simulink model "Pitch_Attitude_Hold"  (R2024b)
settings: Solver=VariableStepAuto  StartTime=0.0  StopTime=35  RelTol=1e-3
undefined symbols (not defined in the file or in its folder): Ki_2, Kp_1, Kp_2
libraries: slpidlib x2
settings Model: Creator=GH-X-ST  LastModifiedBy=GH-X-ST

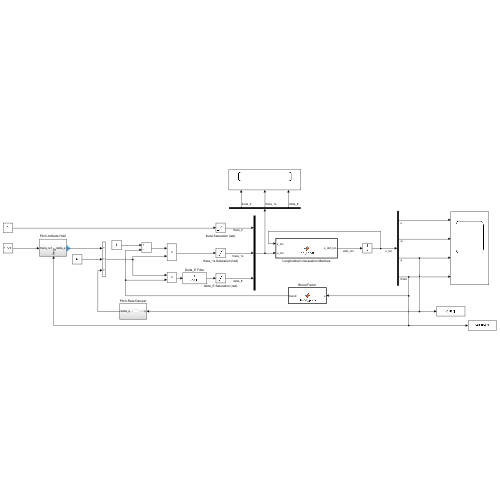
[thumbnail: Simulink's stored preview of the top-level diagram]
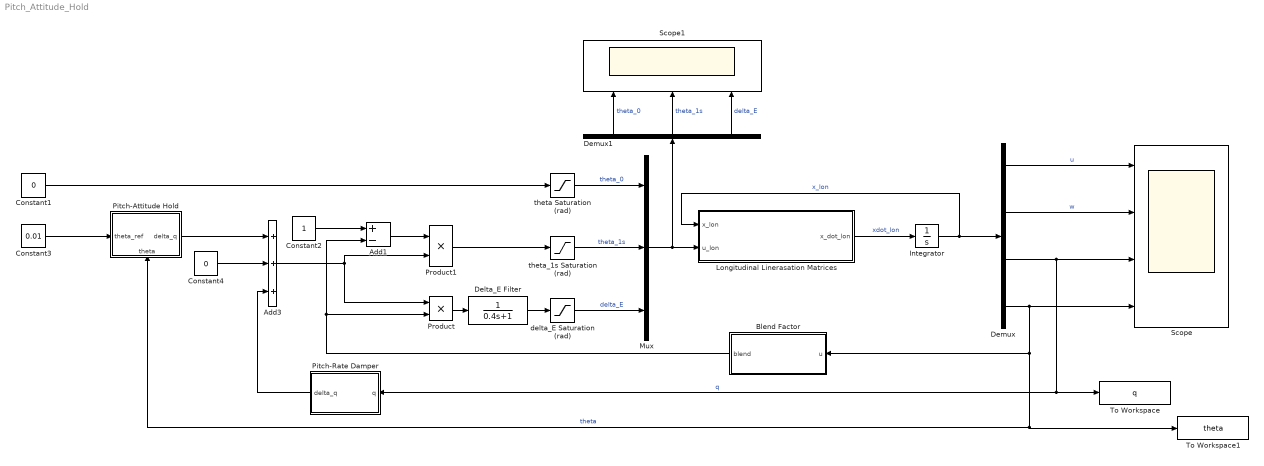
== system Pitch_Attitude_Hold ==
  Add1 : Sum  Inputs=+-
  Add3 : Sum  Inputs=+++
  Blend Factor : MATLAB Function  TreatAsAtomicUnit=on
  Constant1 : Constant  Value=0
  Constant2 : Constant
  Constant3 : Constant  Value=0.01
  Constant4 : Constant  Value=0
  Delta_E Filter : TransferFcn  Denominator=[0.4 1]
  Demux : Demux
  Demux1 : Demux  Outputs=3
  Integrator : Integrator  InitialCondition=[0; 0; 0; 0]
  Longitudinal Linerasation Matrices : MATLAB Function  TreatAsAtomicUnit=on
  Mux : Mux  Inputs=3
  Pitch-Attitude Hold : Subsystem
      settings: PortSchema="{\"entries\":[{\"content\":{\"sides\":[{\"content\":{\"connectorIds\":[\"In1\"]},\"type\":\"ConnectorPlacement.EquallySpacedRectSide\",\"uuid\":\"6ee333b9-9b69-42fd-975a-4580f9624540\"},{\"content\":{\"connectorIds\":[\"Out1\"],\"side\":\"RIGHT\"},\"type\":\"ConnectorPlacement.EquallySpacedRectSide\",\"uuid\":\"6a43d978-a0a5-4636-bfdb-b097e996a039\"},{\"content\":{\"side\":\"TOP\"},\"type\":\"ConnectorPlacement.EquallySpacedRectSide\",\"uuid\":\"00f937d1-ecc9-42d4-adf8-d8f1b79c75a6\"},{\"content\":{\"connectorIds\":[\"In2\"],\"side\":\"BOTTOM\"},\"type\":\"ConnectorPlacement.EquallySpacedRectSide\",\"uuid\":\"809403f9-594f-4491-8a7d-ee0f8643f57e\"}]},\"type\":\"ConnectorPlacement.EquallySpacedConnector\",\"uuid\":\"362aafbc-ebc0-4bb3-8c4e-be284a8bc83f\"}],\"packageUris\":[\"http://schema.mathworks.com/mf0/Connector/R2020b\"],\"version\":\"1.0\"}"
  Pitch-Rate Damper : Subsystem
  Product : Product
  Product1 : Product
  Scope : Scope  NumInputPorts=4
  Scope1 : Scope  NumInputPorts=3
  To Workspace : ToWorkspace  VariableName=q  SaveFormat=Timeseries  SampleTime=-1
  To Workspace1 : ToWorkspace  VariableName=theta  SaveFormat=Timeseries  SampleTime=-1
  delta_E Saturation (rad) : Saturate  UpperLimit=deg2rad(11)  LowerLimit=deg2rad(-11)
  theta Saturation (rad) : Saturate  UpperLimit=deg2rad(20)  LowerLimit=0
  theta_1s Saturation (rad) : Saturate  UpperLimit=deg2rad(6)  LowerLimit=deg2rad(-6)
  wires:
  Longitudinal Linerasation Matrices/1(x_dot_lon) -> Integrator/1  "xdot_lon"
  Integrator/1 -> Longitudinal Linerasation Matrices/1(x_lon), Demux/1  "x_lon"
  Demux/1 -> Scope/1  "u"
  Demux/2 -> Scope/2  "w"
  Demux/3 -> Scope/3, To Workspace/1, Pitch-Rate Damper/1(q)  "q"
  Demux/4 -> To Workspace1/1, Pitch-Attitude Hold/2(theta), Blend Factor/1(u), Scope/4  "theta"
  theta Saturation (rad)/1 -> Mux/1  "theta_0"
  theta_1s Saturation (rad)/1 -> Mux/2  "theta_1s"
  delta_E Saturation (rad)/1 -> Mux/3  "delta_E"
  Blend Factor/1(blend) -> Add1/2, Product/2
  Constant4/1 -> Add3/2
  Pitch-Attitude Hold/1(delta_q) -> Add3/1
  Pitch-Rate Damper/1(delta_q) -> Add3/3
  Add3/1 -> Product/1, Product1/2
  Constant2/1 -> Add1/1
  Add1/1 -> Product1/1
  Mux/1 -> Demux1/1, Longitudinal Linerasation Matrices/2(u_lon)
  Demux1/3 -> Scope1/3  "delta_E"
  Demux1/2 -> Scope1/2  "theta_1s"
  Demux1/1 -> Scope1/1  "theta_0"
  Product/1 -> Delta_E Filter/1
  Product1/1 -> theta_1s Saturation (rad)/1
  Constant1/1 -> theta Saturation (rad)/1
  Constant3/1 -> Pitch-Attitude Hold/1(theta_ref)
  Delta_E Filter/1 -> delta_E Saturation (rad)/1

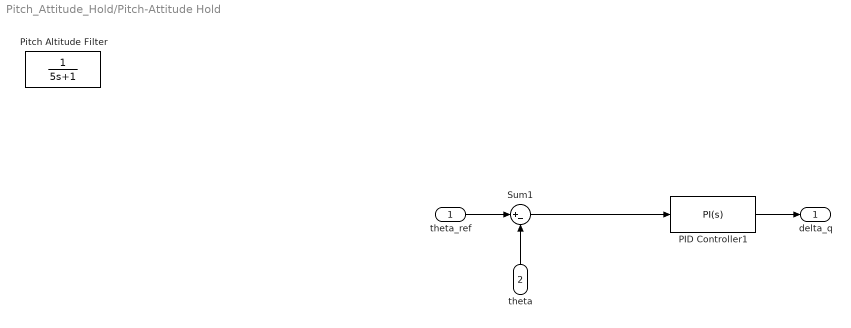
== system Pitch_Attitude_Hold/Pitch-Attitude Hold ==
  theta_ref : Inport
  theta : Inport  Port=2
  PID Controller1 : slpidlib/PID Controller  Controller=PI  Form=Parallel  TimeDomain=Continuous-time  UseExternalTs=off  SampleTime=-1  IntegratorMethod=Forward Euler  FilterMethod=Forward Euler  ControllerParametersSource=internal  P=Kp_2  I=Ki_2  UseKiTs=off  D=0.005  UseExternalDerivativeSource=on  N=100  UseFilter=on  TunerSelectOption=Transfer Function Based (PID Tuner App)  InitialConditionSource=internal  InitialConditionForIntegrator=0  InitialConditionForFilter=0  DifferentiatorICPrevScaledInput=0  ExternalReset=none  TrackingMode=off  Kt=1  LimitOutput=on  SatLimitsSource=internal  UpperSaturationLimit=1  LowerSaturationLimit=-1  LinearizeAsGain=on  AntiWindupMode=none  Kb=1  LimitIntegrator=off  UpperIntegratorSaturationLimit=inf  LowerIntegratorSaturationLimit=-inf  POutMin=[]  POutMax=[]  IOutMin=[]  IOutMax=[]  DOutMin=[]  DOutMax=[]  NOutMin=[]  NOutMax=[]  SumOutMin=[]  SumOutMax=[]  SaturationOutMin=[]  SaturationOutMax=[]  PParamMin=[]  PParamMax=[]  IParamMin=[]  IParamMax=[]  DParamMin=[]  DParamMax=[]  NParamMin=[]  NParamMax=[]  KbParamMin=[]  KbParamMax=[]  KtParamMin=[]  KtParamMax=[]  KbOutMin=[]  KbOutMax=[]  KtOutMin=[]  KtOutMax=[]  IntegratorOutMin=[]  IntegratorOutMax=[]  FilterOutMin=[]  FilterOutMax=[]  SumI1OutMin=[]  SumI1OutMax=[]  SumI2OutMin=[]  SumI2OutMax=[]  SumI3OutMin=[]  SumI3OutMax=[]  SumI4OutMin=[]  SumI4OutMax=[]  SumDOutMin=[]  SumDOutMax=[]  DifferentiatorOutMin=[]  DifferentiatorOutMax=[]  FilterDiffOutCoefMin=[]  FilterDiffOutCoefMax=[]  ReciprocalOutMin=[]  ReciprocalOutMax=[]  SumDenOutMin=[]  SumDenOutMax=[]  SumNumOutMin=[]  SumNumOutMax=[]  DivideOutMin=[]  DivideOutMax=[]  UdiffTsProdOutMin=[]  UdiffTsProdOutMax=[]  NTsProdOutMin=[]  NTsProdOutMax=[]  UintegralTsProdOutMin=[]  UintegralTsProdOutMax=[]  UngainTsProdOutMin=[]  UngainTsProdOutMax=[]  ClampingZeroOutDataTypeStr=Inherit: Inherit via back propagation  ClampingZeroOutMin=[]  ClampingZeroOutMax=[]  FilterDenConstantOutDataTypeStr=Inherit: Inherit via back propagation  FilterDenConstantOutMin=[]  FilterDenConstantOutMax=[]  PCopyOutDataTypeStr=Inherit: Inherit via back propagation  PCopyOutMin=[]  PCopyOutMax=[]  NCopyOutDataTypeStr=Inherit: Inherit via back propagation  NCopyOutMin=[]  NCopyOutMax=[]  IntegratorContinuousStateAttributes=''  IntegratorStateMustResolveToSignalObject=off  IntegratorRTWStateStorageClass=Auto  FilterContinuousStateAttributes=''  FilterStateMustResolveToSignalObject=off  FilterRTWStateStorageClass=Auto  ParallelPVariant=InternalParameters  IdealPVariant=Disabled  IVariant=InternalParameters  DVariant=Disabled  IntegratorVariant=Continuous  SatVariant=Enabled  AWVariant=Passthrough  PCopyVariant=Disabled  TRVariant=Disabled  FdbkBlocksVariant=Forward  IdealPFdbkVariant=Disabled  SatFdbkVariant=Disabled  DerivativeFilterVariant=Disabled  NVariant=Passthrough  NCopyVariant=Disabled_SignalSpec  FilterICVariant=Disabled  IntegratorICVariant=InternalICs  ExternalResetVariant=Disabled  TRSumVariant=Passthrough  SumFdbkVariant=Disabled  SumVariant=Sum_PI  TsampFilterVariant=InternalTs  TsampNgainVariant=Passthrough  TsampIntegralVariant=Disabled_SignalSpec  ExternalSaturationOutDataTypeStr=Inherit: Same as second input  DerivativeSourceVariant=Disabled  PreIntVariant=InternalPreInt
  Pitch Altitude Filter : TransferFcn  Denominator=[5 1]
  Sum1 : Sum  Inputs=|+-
  delta_q : Outport
  wires:
  PID Controller1/1 -> delta_q/1
  theta_ref/1 -> Sum1/1
  theta/1 -> Sum1/2
  Sum1/1 -> PID Controller1/1

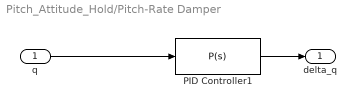
== system Pitch_Attitude_Hold/Pitch-Rate Damper ==
  q : Inport
  PID Controller1 : slpidlib/PID Controller  Controller=P  Form=Parallel  TimeDomain=Continuous-time  UseExternalTs=off  SampleTime=-1  IntegratorMethod=Forward Euler  FilterMethod=Forward Euler  ControllerParametersSource=internal  P=Kp_1  I=0.005  UseKiTs=off  D=0.005  UseExternalDerivativeSource=on  N=100  UseFilter=on  TunerSelectOption=Transfer Function Based (PID Tuner App)  InitialConditionSource=internal  InitialConditionForIntegrator=0  InitialConditionForFilter=0  DifferentiatorICPrevScaledInput=0  ExternalReset=none  TrackingMode=off  Kt=1  LimitOutput=on  SatLimitsSource=internal  UpperSaturationLimit=1  LowerSaturationLimit=-1  LinearizeAsGain=on  AntiWindupMode=none  Kb=1  LimitIntegrator=off  UpperIntegratorSaturationLimit=inf  LowerIntegratorSaturationLimit=-inf  POutMin=[]  POutMax=[]  IOutMin=[]  IOutMax=[]  DOutMin=[]  DOutMax=[]  NOutMin=[]  NOutMax=[]  SumOutMin=[]  SumOutMax=[]  SaturationOutMin=[]  SaturationOutMax=[]  PParamMin=[]  PParamMax=[]  IParamMin=[]  IParamMax=[]  DParamMin=[]  DParamMax=[]  NParamMin=[]  NParamMax=[]  KbParamMin=[]  KbParamMax=[]  KtParamMin=[]  KtParamMax=[]  KbOutMin=[]  KbOutMax=[]  KtOutMin=[]  KtOutMax=[]  IntegratorOutMin=[]  IntegratorOutMax=[]  FilterOutMin=[]  FilterOutMax=[]  SumI1OutMin=[]  SumI1OutMax=[]  SumI2OutMin=[]  SumI2OutMax=[]  SumI3OutMin=[]  SumI3OutMax=[]  SumI4OutMin=[]  SumI4OutMax=[]  SumDOutMin=[]  SumDOutMax=[]  DifferentiatorOutMin=[]  DifferentiatorOutMax=[]  FilterDiffOutCoefMin=[]  FilterDiffOutCoefMax=[]  ReciprocalOutMin=[]  ReciprocalOutMax=[]  SumDenOutMin=[]  SumDenOutMax=[]  SumNumOutMin=[]  SumNumOutMax=[]  DivideOutMin=[]  DivideOutMax=[]  UdiffTsProdOutMin=[]  UdiffTsProdOutMax=[]  NTsProdOutMin=[]  NTsProdOutMax=[]  UintegralTsProdOutMin=[]  UintegralTsProdOutMax=[]  UngainTsProdOutMin=[]  UngainTsProdOutMax=[]  ClampingZeroOutDataTypeStr=Inherit: Inherit via back propagation  ClampingZeroOutMin=[]  ClampingZeroOutMax=[]  FilterDenConstantOutDataTypeStr=Inherit: Inherit via back propagation  FilterDenConstantOutMin=[]  FilterDenConstantOutMax=[]  PCopyOutDataTypeStr=Inherit: Inherit via back propagation  PCopyOutMin=[]  PCopyOutMax=[]  NCopyOutDataTypeStr=Inherit: Inherit via back propagation  NCopyOutMin=[]  NCopyOutMax=[]  IntegratorContinuousStateAttributes=''  IntegratorStateMustResolveToSignalObject=off  IntegratorRTWStateStorageClass=Auto  FilterContinuousStateAttributes=''  FilterStateMustResolveToSignalObject=off  FilterRTWStateStorageClass=Auto  ParallelPVariant=InternalParameters  IdealPVariant=Disabled  IVariant=Disabled  DVariant=Disabled  IntegratorVariant=Disabled  SatVariant=Enabled  AWVariant=Disabled  PCopyVariant=Disabled  TRVariant=Disabled  FdbkBlocksVariant=Forward  IdealPFdbkVariant=Disabled  SatFdbkVariant=Disabled  DerivativeFilterVariant=Disabled  NVariant=Passthrough  NCopyVariant=Disabled_SignalSpec  FilterICVariant=Disabled  IntegratorICVariant=Disabled  ExternalResetVariant=Disabled  TRSumVariant=Passthrough  SumFdbkVariant=Disabled  SumVariant=Passthrough_P  TsampFilterVariant=InternalTs  TsampNgainVariant=Passthrough  TsampIntegralVariant=Disabled_SignalSpec  ExternalSaturationOutDataTypeStr=Inherit: Same as second input  DerivativeSourceVariant=Disabled  PreIntVariant=InternalPreInt
  delta_q : Outport
  wires:
  PID Controller1/1 -> delta_q/1
  q/1 -> PID Controller1/1

== matlab function Pitch_Attitude_Hold/Longitudinal Linerasation Matrices ==
  data: x_lon input; u_lon input; x_dot_lon output
function x_dot_lon = Lon_linear(x_lon, u_lon)
% Author:
%   Hanchen Li (hl3422@ic.ac.uk)
%
% Inputs:
%   x_lon     - [u, w, q, theta]
%   u         - Forward velocity (m/s)
%   w         - Vertical velocity (m/s)
%   q         - Pitch rate (rad/s)
%   theta     - Euler pitch angle (rad)
%
%   u_lon     - [theta_0, theta_1s, delta_E]
%   theta_0   - Average rotor collective (rad)
%   theta_1s  - Longitudinal cyclic (rad)
%   delta_E   - Elevator deflection (rad)
%
% Outputs:
%   x_dot_lon - [u_dot, w_dot, q_dot, theta_dot]

%% 0 Extract Parameters
u     = x_lon(1);
% w     = x_lon(2);
% q     = x_lon(3);
% theta = x_lon(4);

% theta_0 = u_lon(1);
% theta_1s = u_lon(2);
% delta_E = u_lon(3);

%% 1 Initial parameters
U = [0; 20; 40; 60; 72.0222222]; % 5 break-points

A_lon_all = cat(3,...
[-0.00723802383207751	-1.35323092947785e-20	-0.766629187912504	-9.80664998365558;
-3.64153152077051e-10	-0.626783991819480	0	0;
0.000872483038786669	1.53518643043251e-21	0.0942177477514433	0;
0	0	1	0],...
[-0.0112549858980772	0.0371668055628924	-1.18927896465665	-9.80422222650819;
-0.133476123611587	-1.29584894245305	20.8981012783838	-0.0361550902372443;
0.0229512851532743	0.0212311520956117	-1.57834195971935	0;
0	0	0.999823172370649	0],...
[-0.00894644618554263	0.0320555490226915	-1.19654303458228	-9.78886874671681;
0.0177938328871363	-2.75625714952099	41.9669994347238	0.0565348232672847;
0.00544480361520019	0.0390031290231026	-1.68547625422026	0;
0	0	0.999701937133157	0],...
[-0.00115522776185373	0.0138477446845475	-1.25249222634898	-9.78189512322418;
0.129681745697496	-2.84658770249635	62.0992998719228	-0.370385725787514;
-6.84962619262734e-05	0.0554454638454316	-1.71412794300992	0;
0	0	0.999829013944947	0],...
[0.00198907487199834	0.00124807180451603	-1.31545814391634	-9.77936080280246;
0.208959151679622	-2.91377790533787	74.4525040940847	-0.690902155824347;
-0.00261903529268842	0.0663122914709030	-1.76288467057787	0;
0	0	0.999876306745786	0]);

B_lon_all = cat(3,...
[-2.41065865317012e-18	-5.17979000748556	0;
-111.654787649114	0	0;
2.95095583193773e-19	0.636589574236795	0;
0	0	0],...
[3.61243491647048	-7.51807669482774	0.00519991275444581;
-211.546063860615	-28.3860279697912	-0.718873847311841;
-3.72624202744466	-15.9950728844985	-0.301829974738856;
0	0	0],...
[-2.10906781602821	-8.34051477693776	-0.000966485101117076;
-228.851268194816	-60.5903363544424	-2.65783402805475;
-7.49489399091787	-17.9234263896394	-1.11495618916578;
0	0	0],...
[-6.26132311908841	-9.73615029140097	0;
-245.122010910137	-92.4433695878246	-6.00187247789208;
-13.3651657046107	-20.4991398778183	-2.51787921575724;
0	0	0],...
[-9.36734534820370	-11.2809889940346	0;
-257.948569477389	-112.985439522211	-8.64803218389554;
-16.7725921688728	-22.1441400308729	-3.62798452869815;
0	0	0]);

%% 2 Vectorised interpolation
% method = 'pchip';

% A_lon =  squeeze( interp1(U, permute(A_lon_all,[3 1 2]), u, method, 'extrap') );
% B_lon =  squeeze( interp1(U, permute(B_lon_all,[3 1 2]), u, method, 'extrap') );

A_lon = ...
[-0.00723802383207751	-1.35323092947785e-20	-0.766629187912504	-9.80664998365558;
-3.64153152077051e-10	-0.626783991819480	0	0;
0.000872483038786669	1.53518643043251e-21	0.0942177477514433	0;
0	0	1	0];

B_lon = ...
[-2.41065865317012e-18	-5.17979000748556	0;
-111.654787649114	0	0;
2.95095583193773e-19	0.636589574236795	0;
0	0	0];

%% 3 Output
x_dot_lon = A_lon * x_lon + B_lon * u_lon;

end

== matlab function Pitch_Attitude_Hold/Blend Factor ==
  data: blend output; u input
function blend = Blend_pitch(u)
% Author:
%   Hanchen Li (hl3422@ic.ac.uk)
%
% Inputs:
%   u         - Forward velocity (m/s)
%
% Outputs:
%   blend     - blend factor

%% 1 Decide blend factor

if abs(u) < 1e-4

    blend = 0;

elseif abs(u) < 90.3

    blend = u / (90.3 / 0.8);

else

    blend = 0.8;

end

end
